simulink model "SMC_Example"  (R2021b)
settings: Solver=ode1  StartTime=0.0  StopTime=5  FixedStep=0.001  RelTol=1e-3
PreLoadFcn:
  | run('Example_init.m')
values from neighbouring files (symbols this model uses):
  A = BWB.lat.A    [SMC_Example_init.m]
  ADPT = 0    [SMC_Example_init.m]
  Ao = At    [SMCDesign_init.m]    (also in SMCDesign_initIA.m)
  B = BWB.lat.B    [SMC_Example_init.m]
  Bo = Bv    [SMCDesign_init.m]    (also in SMCDesign_initIA.m)
  C = eye(n)    [SMC_Example_init.m]
  C0 = 0    [SMC_Example_init.m]
  Cc = [1 0 0 0 ... (first row only)    [SMC_Example_init.m]
  Co = Ct    [SMCDesign_init.m]    (also in SMCDesign_initIA.m)
  D = zeros(p,m)    [SMC_Example_init.m]
  delta = 0.01    [SMC_Example_init.m]
  deltao = 0.01    [SMC_Example_init.m]
  FR = -eye(ll)    [SMC_Example_init.m]
  K0 = 0    [SMC_Example_init.m]
  L = L*Tr    [SMCDesign_init.m]    (also in SMCDesign_initIA.m = L*TT; contliaCA.m = -inv(Lam)*(S*AT-Phi*S))
  Lam_inv = inv(Lam)    [SMCDesign_init.m]    (also in SMCDesign_initIA.m)
  Lr = -inv(Lam)*(Phi*Sr+Snew(:,1:pp))    [contliaCA.m]
  Lrdot = inv(Lam)*Sr    [contliaCA.m]
  P = lyap(Phi',eye(mm))    [contliaCA.m]
  PC = 1    [SMC_Example_init.m]
  PK = 1    [SMC_Example_init.m]
  rho = 5    [SMC_Example_init.m]
  rhoo = 15    [SMC_Example_init.m]
  S = S*Tr    [SMCDesign_init.m]    (also in SMCDesign_initIA.m = S*TT; lqcfCA.m = [M eye(mm)]*Tr)
  Sr = -Snew(:,nn+pp-mm+1:nn+pp)*inv(Br'*inv(A11s)*A12a)*Br'*inv(A11s)*Br    [contliaCA.m]
  To_inv = inv(Tr)    [SMCDesign_init.m]    (also in SMCDesign_initIA.m)
  x0 = zeros(1,n)    [SMC_Example_init.m]
  z0 = zeros(1,n)    [SMC_Example_init.m]
undefined symbols (not defined in the file or in its folder): CA, F, G, Gl, Gn, P2
libraries: SMC x2
settings Model: Creator=lev201  LastModifiedBy=w.schwamm
settings SolverCC: AlgebraicLoopSolver=TrustRegion
settings DataIOCC: ReturnWorkspaceOutputs=off
settings DebuggingCC: SFMachineParentedDataDiag=warning  ArithmeticOperatorsInVariantConditions=warning
settings SFSimCC: SimUseLocalCustomCode=off  CustomCodeUndefinedFunction=UseInterfaceOnly
settings RTWCC: RTWUseLocalCustomCode=off

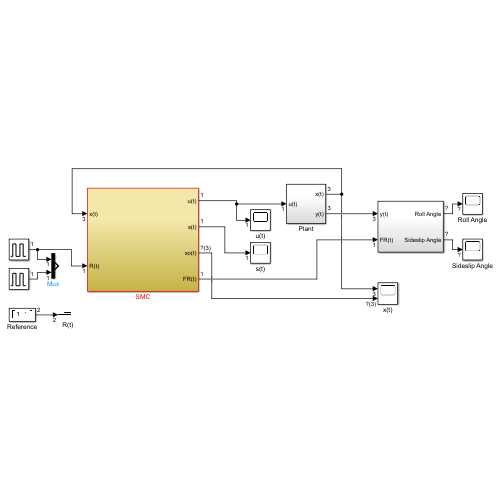
[thumbnail: Simulink's stored preview of the top-level diagram]
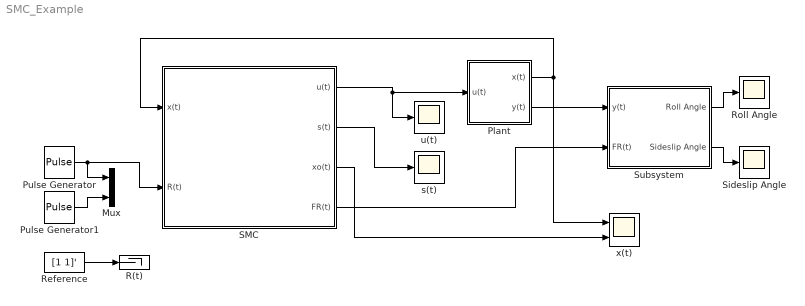
== system SMC_Example ==
  Mux : Mux  Inputs=2
  Plant : Subsystem
  Pulse Generator : DiscretePulseGenerator  PulseType=Time based  Period=20  PulseWidth=50
  Pulse Generator1 : DiscretePulseGenerator  PulseType=Time based  Period=20  PulseWidth=50  PhaseDelay=10
  R(t) : Terminator
  Reference : Constant  Value=[1 1]'
  Roll Angle : Scope
  SMC : Subsystem
  Sideslip Angle : Scope
  Subsystem : Subsystem
  s(t) : Scope
  u(t) : Scope
  x(t) : Scope  NumInputPorts=2
  wires:
  Plant/2(y(t)) -> Subsystem/1(y(t))
  SMC/1(u(t)) -> u(t)/1, Plant/1(u(t))
  Subsystem/1(Roll Angle) -> Roll Angle/1
  Subsystem/2(Sideslip Angle) -> Sideslip Angle/1
  Pulse Generator/1 -> SMC/2(R(t)), Mux/1
  Pulse Generator1/1 -> Mux/2
  SMC/2(s(t)) -> s(t)/1
  Plant/1(x(t)) -> x(t)/1, SMC/1(x(t))
  Reference/1 -> R(t)/1
  SMC/3(xo(t)) -> x(t)/2
  SMC/4(FR(t)) -> Subsystem/2(FR(t))

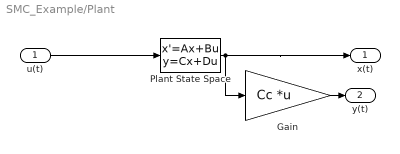
== system SMC_Example/Plant ==
  u(t) : Inport
  Gain : Gain  Gain=Cc  Multiplication=Matrix(K*u) (u vector)
  Plant State Space : StateSpace  A=A  B=B  C=C  D=D  InitialCondition=x0
  x(t) : Outport  VectorParamsAs1DForOutWhenUnconnected=off
  y(t) : Outport  Port=2  VectorParamsAs1DForOutWhenUnconnected=off
  wires:
  u(t)/1 -> Plant State Space/1
  Plant State Space/1 -> Gain/1, x(t)/1
  Gain/1 -> y(t)/1

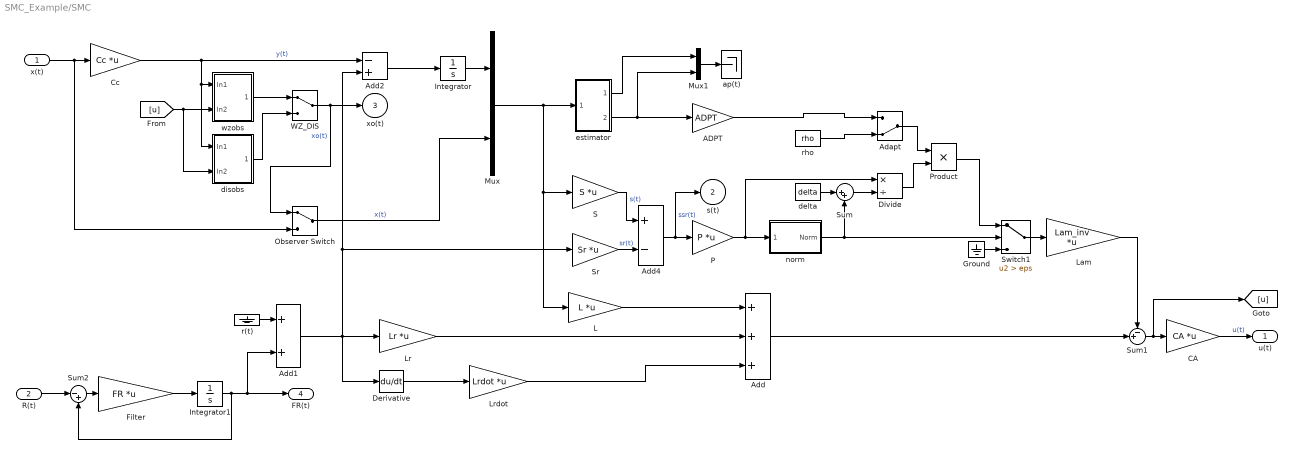
== system SMC_Example/SMC ==
  x(t) : Inport
  R(t) : Inport  Port=2
  ADPT : Gain  Gain=ADPT
  Adapt : ManualSwitch  CurrentSetting=0
  Add : Sum  Inputs=+++
  Add1 : Sum
  Add2 : Sum  Inputs=-+
  Add4 : Sum  Inputs=+-
  CA : Gain  Gain=CA  Multiplication=Matrix(K*u) (u vector)
  Cc : Gain  Gain=Cc  Multiplication=Matrix(K*u) (u vector)
  Derivative : Derivative
  Divide : Product  Inputs=*/
  Filter : Gain  Gain=FR  Multiplication=Matrix(K*u) (u vector)
  Ground : Ground
  Integrator : Integrator
  Integrator1 : Integrator
  L : Gain  Gain=L  Multiplication=Matrix(K*u) (u vector)
  Lam : Gain  Gain=Lam_inv  Multiplication=Matrix(K*u) (u vector)
  Lr : Gain  Gain=Lr  Multiplication=Matrix(K*u) (u vector)
  Lrdot : Gain  Gain=Lrdot  Multiplication=Matrix(K*u) (u vector)
  Mux : Mux  Inputs=2
  Mux1 : Mux  Inputs=2
  Observer Switch : ManualSwitch
  P : Gain  Gain=P  Multiplication=Matrix(K*u) (u vector)
  Product : Product
  S : Gain  Gain=S  Multiplication=Matrix(K*u) (u vector)
  Sr : Gain  Gain=Sr  Multiplication=Matrix(K*u) (u vector)
  Sum : Sum  Inputs=|++
  Sum1 : Sum  Inputs=-+|
  Sum2 : Sum  Inputs=|-+
  Switch1 : Switch  Criteria=u2 > Threshold  Threshold=eps  ZeroCross=off
  WZ_DIS : ManualSwitch
  ap(t) : Terminator
  delta : Constant  Value=delta
  disobs : Subsystem
  estimator : Subsystem
  norm : Subsystem
  r(t) : Ground
  rho : Constant  Value=rho
  wzobs : Subsystem
  u(t) : Outport  VectorParamsAs1DForOutWhenUnconnected=off
  s(t) : Outport  Port=2
  xo(t) : Outport  Port=3
  FR(t) : Outport  Port=4
  wires:
  Cc/1 -> disobs/1(In1), wzobs/1(In1), Add2/1  "y(t)"
  x(t)/1 -> Cc/1, Observer Switch/2
  WZ_DIS/1 -> xo(t)/1, Observer Switch/1  "xo(t)"
  wzobs/1(Out1) -> WZ_DIS/1
  disobs/1(Out1) -> WZ_DIS/2
  [u] -> wzobs/2(In2), disobs/2(In2)
  Observer Switch/1 -> Mux/2  "x(t)"
  Lrdot/1 -> Add/3
  Derivative/1 -> Lrdot/1
  S/1 -> Add4/1  "s(t)"
  Sr/1 -> Add4/2  "sr(t)"
  Lam/1 -> Sum1/1
  Product/1 -> Switch1/1
  ADPT/1 -> Adapt/1
  rho/1 -> Adapt/2
  Adapt/1 -> Product/1
  estimator/2(rho) -> Mux1/2, ADPT/1
  Mux1/1 -> ap(t)/1
  estimator/1(est-par) -> Mux1/1
  Switch1/1 -> Lam/1
  Ground/1 -> Switch1/3
  Filter/1 -> Integrator1/1
  Integrator1/1 -> Add1/2, FR(t)/1, Sum2/2
  Sum2/1 -> Filter/1
  R(t)/1 -> Sum2/1
  Add1/1 -> Derivative/1, Lr/1, Add2/2, Sr/1
  r(t)/1 -> Add1/1
  Mux/1 -> estimator/1(x(t)), S/1, L/1
  Lr/1 -> Add/2
  delta/1 -> Sum/1
  Sum/1 -> Divide/2
  L/1 -> Add/1
  Integrator/1 -> Mux/1
  Add2/1 -> Integrator/1
  Add4/1 -> P/1, s(t)/1  "ssr(t)"
  Sum1/1 -> CA/1, [u]
  CA/1 -> u(t)/1  "u(t)"
  Divide/1 -> Product/2
  P/1 -> norm/1(Vector), Divide/1
  norm/1(Norm) -> Switch1/2, Sum/2
  Add/1 -> Sum1/2

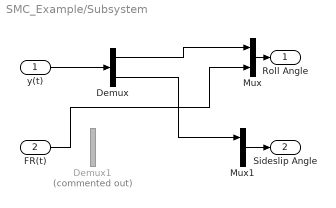
== system SMC_Example/Subsystem ==
  y(t) : Inport
  FR(t) : Inport  Port=2
  Demux : Demux  Outputs=2
  Demux1 : Demux  Commented=on  Outputs=2
  Mux : Mux  Inputs=2
  Mux1 : Mux  Inputs=2
  Roll Angle : Outport  VectorParamsAs1DForOutWhenUnconnected=off
  Sideslip Angle : Outport  Port=2  VectorParamsAs1DForOutWhenUnconnected=off
  wires:
  y(t)/1 -> Demux/1
  Demux/1 -> Mux/1
  Mux/1 -> Roll Angle/1
  Mux1/1 -> Sideslip Angle/1
  Demux/2 -> Mux1/1
  FR(t)/1 -> Mux/2

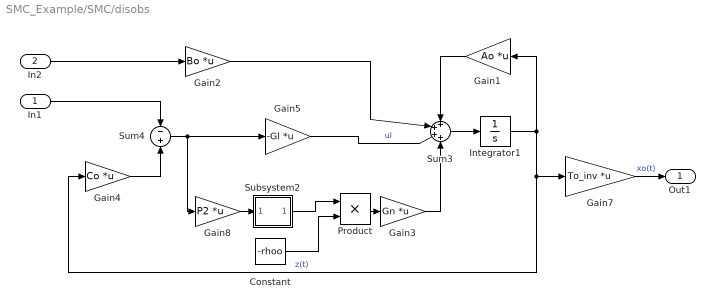
== system SMC_Example/SMC/disobs ==
  In1 : Inport
  In2 : Inport  Port=2
  Constant : Constant  Value=-rhoo  SampleTime=-1
  Gain1 : Gain  Gain=Ao  Multiplication=Matrix(K*u)
  Gain2 : Gain  Gain=Bo  Multiplication=Matrix(K*u)
  Gain3 : Gain  Gain=Gn  Multiplication=Matrix(K*u)
  Gain4 : Gain  Gain=Co  Multiplication=Matrix(K*u)
  Gain5 : Gain  Gain=-Gl  Multiplication=Matrix(K*u)
  Gain7 : Gain  Gain=To_inv  Multiplication=Matrix(K*u)
  Gain8 : Gain  Gain=P2  Multiplication=Matrix(K*u)
  Integrator1 : Integrator  InitialCondition=z0
  Product : Product
  Subsystem2 : Subsystem  mask{delta=deltao}
      mask prompts: delta "Unit vector delta:"
      mask Display: disp('UnV')
  Sum3 : Sum  Inputs=++++
  Sum4 : Sum  Inputs=-+
  Out1 : Outport
  wires:
  Subsystem2/1(Out1) -> Product/1
  Product/1 -> Gain3/1
  Constant/1 -> Product/2
  Gain7/1 -> Out1/1  "xo(t)"
  Gain5/1 -> Sum3/3  "ul"
  Sum4/1 -> Gain5/1, Gain8/1
  Integrator1/1 -> Gain1/1, Gain7/1, Gain4/1  "z(t)"
  Gain4/1 -> Sum4/2
  Gain2/1 -> Sum3/2
  Gain8/1 -> Subsystem2/1(In1)
  Gain3/1 -> Sum3/4
  Gain1/1 -> Sum3/1
  Sum3/1 -> Integrator1/1
  In2/1 -> Gain2/1
  In1/1 -> Sum4/1

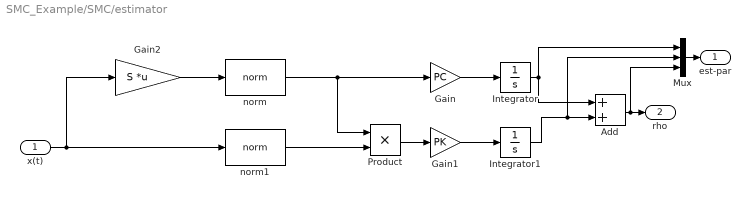
== system SMC_Example/SMC/estimator ==
  x(t) : Inport
  Add : Sum
  Gain : Gain  Gain=PC
  Gain1 : Gain  Gain=PK
  Gain2 : Gain  Gain=S  Multiplication=Matrix(K*u) (u vector)
  Integrator : Integrator  InitialCondition=C0
  Integrator1 : Integrator  InitialCondition=K0
  Mux : Mux  Inputs=3
  Product : Product
  norm : SMC/SMC/norm  SystemSampleTime=-1  VariantActivationTime=update diagram  Latency=0  AutoFrameSizeCalculation=off
      settings: SourceProductName=Sliding Mode Control Toolbox
  norm1 : SMC/SMC/norm  SystemSampleTime=-1  VariantActivationTime=update diagram  Latency=0  AutoFrameSizeCalculation=off
      settings: SourceProductName=Sliding Mode Control Toolbox
  est-par : Outport  VectorParamsAs1DForOutWhenUnconnected=off
  rho : Outport  Port=2  VectorParamsAs1DForOutWhenUnconnected=off
  wires:
  Mux/1 -> est-par/1
  Gain2/1 -> norm/1
  Integrator1/1 -> Add/2, Mux/2
  Add/1 -> rho/1, Mux/3
  Gain1/1 -> Integrator1/1
  Product/1 -> Gain1/1
  norm1/1 -> Product/2
  x(t)/1 -> Gain2/1, norm1/1
  norm/1 -> Gain/1, Product/1
  Integrator/1 -> Mux/1, Add/1
  Gain/1 -> Integrator/1

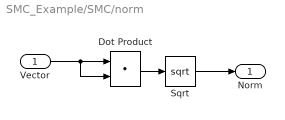
== system SMC_Example/SMC/norm ==
  Vector : Inport
  Dot Product : DotProduct  InputSameDT=on  OutDataTypeStr=Inherit: Inherit via internal rule
  Sqrt : Sqrt  SaturateOnIntegerOverflow=on
  Norm : Outport  VectorParamsAs1DForOutWhenUnconnected=off
  wires:
  Sqrt/1 -> Norm/1
  Vector/1 -> Dot Product/1, Dot Product/2
  Dot Product/1 -> Sqrt/1

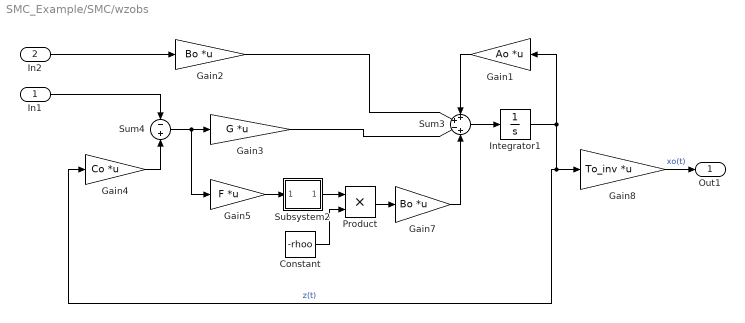
== system SMC_Example/SMC/wzobs ==
  In1 : Inport
  In2 : Inport  Port=2
  Constant : Constant  Value=-rhoo  SampleTime=-1
  Gain1 : Gain  Gain=Ao  Multiplication=Matrix(K*u) (u vector)
  Gain2 : Gain  Gain=Bo  Multiplication=Matrix(K*u) (u vector)
  Gain3 : Gain  Gain=G  Multiplication=Matrix(K*u) (u vector)
  Gain4 : Gain  Gain=Co  Multiplication=Matrix(K*u) (u vector)
  Gain5 : Gain  Gain=F  Multiplication=Matrix(K*u) (u vector)
  Gain7 : Gain  Gain=Bo  Multiplication=Matrix(K*u) (u vector)
  Gain8 : Gain  Gain=To_inv  Multiplication=Matrix(K*u) (u vector)
  Integrator1 : Integrator  InitialCondition=z0
  Product : Product
  Subsystem2 : Subsystem  mask{delta=deltao}
      mask prompts: delta "Unit vector delta:"
      mask Display: disp('UnV')
  Sum3 : Sum  Inputs=++-+
  Sum4 : Sum  Inputs=-+
  Out1 : Outport
  wires:
  Gain8/1 -> Out1/1  "xo(t)"
  Constant/1 -> Product/2
  In1/1 -> Sum4/1
  In2/1 -> Gain2/1
  Sum3/1 -> Integrator1/1
  Gain1/1 -> Sum3/1
  Gain3/1 -> Sum3/3
  Gain7/1 -> Sum3/4
  Subsystem2/1(Out1) -> Product/1
  Gain5/1 -> Subsystem2/1(In1)
  Product/1 -> Gain7/1
  Gain2/1 -> Sum3/2
  Gain4/1 -> Sum4/2
  Integrator1/1 -> Gain1/1, Gain8/1, Gain4/1  "z(t)"
  Sum4/1 -> Gain3/1, Gain5/1

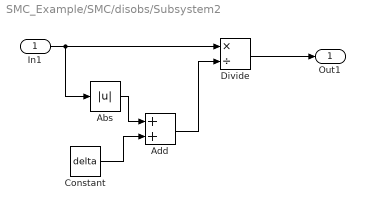
== system SMC_Example/SMC/disobs/Subsystem2 ==
  In1 : Inport
  Abs : Abs  ZeroCross=off
  Add : Sum
  Constant : Constant  Value=delta  SampleTime=-1
  Divide : Product  Inputs=*/
  Out1 : Outport
  wires:
  Constant/1 -> Add/2
  Add/1 -> Divide/2
  Abs/1 -> Add/1
  Divide/1 -> Out1/1
  In1/1 -> Divide/1, Abs/1

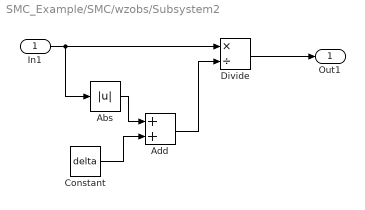
== system SMC_Example/SMC/wzobs/Subsystem2 ==
  In1 : Inport
  Abs : Abs  ZeroCross=off
  Add : Sum
  Constant : Constant  Value=delta  SampleTime=-1
  Divide : Product  Inputs=*/
  Out1 : Outport
  wires:
  In1/1 -> Abs/1, Divide/1
  Divide/1 -> Out1/1
  Abs/1 -> Add/1
  Add/1 -> Divide/2
  Constant/1 -> Add/2
